simulink library "MathLib"  (R2016b)
settings: Solver=VariableStepAuto  StartTime=0.0  StopTime=10.0  RelTol=1e-3
settings Model: Creator=Administrator  LastModifiedBy=Administrator

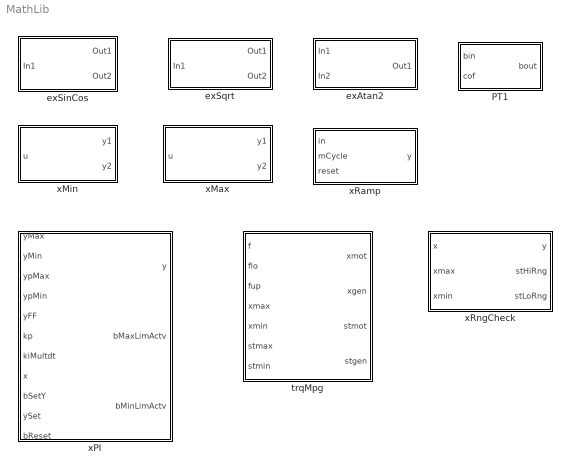
== system MathLib ==
  PT1 : Subsystem
      settings: RTWFcnNameOpts=Use subsystem name  RTWFileNameOpts=Use subsystem name
  exAtan2 : Subsystem
      mask help:
      | tan(theta) = yAxis/xAxis
      | theta: [0 65536) --> [0 360)
      mask Display:
      | disp('atan2 in C');
      | port_label('input',1,'yAxis');
      | port_label('input',2,'xAxis');
      | port_label('output',1,'theta');
  exSinCos : Subsystem
      mask help:
      | x: [0 65536) -->[0 360)
      | sin: [-32767 32767] -->[-1 1]
      | cos: [-32767 32767] -->[-1 1]
      mask Display:
      | disp('sincos in C');
      | port_label('input',1,'x');
      | port_label('output',1,'sinx');
      | port_label('output',2,'cosx');
  exSqrt : Subsystem
      mask help: x=0 when x<0
      mask Display:
      | disp('sqrt in C');
      | port_label('input',1,'x');
      | port_label('output',1,'sqrtx');
      | port_label('output',2,'1/sqrtx');
  trqMpg : MATLAB Function  TreatAsAtomicUnit=on
  xMax : MATLAB Function  TreatAsAtomicUnit=on
  xMin : MATLAB Function  TreatAsAtomicUnit=on
  xPI : MATLAB Function  TreatAsAtomicUnit=on
  xRamp : MATLAB Function  TreatAsAtomicUnit=on
  xRngCheck : MATLAB Function  TreatAsAtomicUnit=on

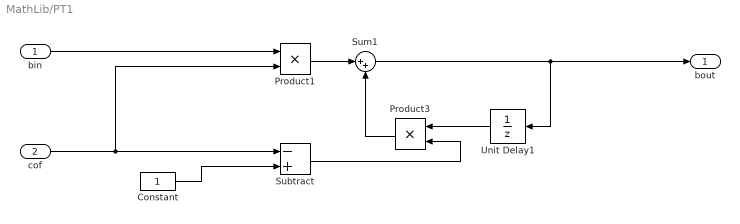
== system MathLib/PT1 ==
  bin : Inport
  cof : Inport  Port=2
  Constant : Constant  OutDataTypeStr=single
  Product1 : Product  RndMeth=Zero  OutDataTypeStr=Inherit: Same as first input
  Product3 : Product  RndMeth=Zero  OutDataTypeStr=Inherit: Same as first input
  Subtract : Sum  Inputs=-+  OutDataTypeStr=Inherit: Same as first input
  Sum1 : Sum  Inputs=|++  OutDataTypeStr=Inherit: Same as first input
  Unit Delay1 : UnitDelay  SampleTime=-1
  bout : Outport
  wires:
  Subtract/1 -> Product3/2
  Sum1/1 -> Unit Delay1/1, bout/1
  cof/1 -> Product1/2, Subtract/1
  Constant/1 -> Subtract/2
  bin/1 -> Product1/1
  Product1/1 -> Sum1/1
  Unit Delay1/1 -> Product3/1
  Product3/1 -> Sum1/2

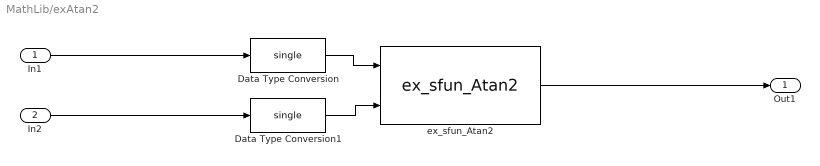
== system MathLib/exAtan2 ==
  In1 : Inport
  In2 : Inport  Port=2
  Data Type Conversion : DataTypeConversion  OutDataTypeStr=single
  Data Type Conversion1 : DataTypeConversion  OutDataTypeStr=single
  ex_sfun_Atan2 : S-Function  FunctionName=ex_sfun_Atan2  SFunctionDeploymentMode=off  EnableBusSupport=off  mask(Legacy Function){SFunctionSpec=void Atan2Shell(single u1,single u2,uint16 y1[1]), ShowSpec=on}
      mask prompts: ShowSpec "Display function specification"
      mask help:
      | This block allows you to call the legacy functions specified by the following Legacy Code Tool definition:
      | def.SFunctionName = 'ex_sfun_Atan2';
      | def.OutputFcnSpec = 'void Atan2Shell(single u1,single u2,uint16 y1[1])';
      | def.HeaderFiles = {'C2SfunShell.h', 'typedefs.h', 'LIB_Atan2.h', 'LIB_SinCosCalc.h', 'LIB_SqrtCalc.h'};
      | def.SourceFiles = {'C2SfunShell.c', 'LIB_Atan2.c', 'LIB_SinCosCalc.c', 'LIB_SqrtCalc.c'};
      mask Help: <p>This block was generated automatically by the Legacy Code Tool. For detailed help on this tool, call<a href="matlab:legacy_code('help')"> legacy_code('help')</a>.</p>
      mask Callback ShowSpec:
      | if strcmp(get_param(gcbh, 'ShowSpec'), 'on')
      |   set_param(gcbh, 'MaskDisplay', sprintf('fprintf(''%s'');', get_param(gcbh, 'SFunctionSpec')));
      | else
      |   set_param(gcbh, 'MaskDisplay', sprintf('fprintf(''%s'');', get_param(gcbh, 'FunctionName')));
      | end
      mask Display: fprintf('void Atan2Shell(single u1,single u2,uint16 y1[1])');
  Out1 : Outport
  wires:
  Data Type Conversion1/1 -> ex_sfun_Atan2/2
  Data Type Conversion/1 -> ex_sfun_Atan2/1
  In1/1 -> Data Type Conversion/1
  ex_sfun_Atan2/1 -> Out1/1
  In2/1 -> Data Type Conversion1/1

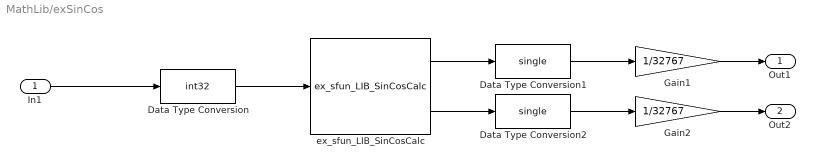
== system MathLib/exSinCos ==
  In1 : Inport
  Data Type Conversion : DataTypeConversion  OutDataTypeStr=int32
  Data Type Conversion1 : DataTypeConversion  OutDataTypeStr=single
  Data Type Conversion2 : DataTypeConversion  OutDataTypeStr=single
  Gain1 : Gain  Gain=1/32767
  Gain2 : Gain  Gain=1/32767
  ex_sfun_LIB_SinCosCalc : S-Function  FunctionName=ex_sfun_LIB_SinCosCalc  SFunctionDeploymentMode=off  EnableBusSupport=off  mask(Legacy Function){SFunctionSpec=void SinCosShell(int32 u1,int16 y1[1],int16 y2[1]), ShowSpec=on}
      mask prompts: ShowSpec "Display function specification"
      mask help:
      | This block allows you to call the legacy functions specified by the following Legacy Code Tool definition:
      | def.SFunctionName = 'ex_sfun_LIB_SinCosCalc';
      | def.OutputFcnSpec = 'void SinCosShell(int32 u1,int16 y1[1],int16 y2[1])';
      | def.HeaderFiles = {'C2SfunShell.h', 'typedefs.h', 'LIB_Atan2.h', 'LIB_SinCosCalc.h', 'LIB_SqrtCalc.h'};
      | def.SourceFiles = {'C2SfunShell.c', 'LIB_Atan2.c', 'LIB_SinCosCalc.c', 'LIB_SqrtCalc.c'};
      mask Help: <p>This block was generated automatically by the Legacy Code Tool. For detailed help on this tool, call<a href="matlab:legacy_code('help')"> legacy_code('help')</a>.</p>
      mask Callback ShowSpec:
      | if strcmp(get_param(gcbh, 'ShowSpec'), 'on')
      |   set_param(gcbh, 'MaskDisplay', sprintf('fprintf(''%s'');', get_param(gcbh, 'SFunctionSpec')));
      | else
      |   set_param(gcbh, 'MaskDisplay', sprintf('fprintf(''%s'');', get_param(gcbh, 'FunctionName')));
      | end
      mask Display: fprintf('void SinCosShell(int32 u1,int16 y1[1],int16 y2[1])');
  Out1 : Outport
  Out2 : Outport  Port=2
  wires:
  Gain1/1 -> Out1/1
  ex_sfun_LIB_SinCosCalc/1 -> Data Type Conversion1/1
  Data Type Conversion1/1 -> Gain1/1
  Data Type Conversion/1 -> ex_sfun_LIB_SinCosCalc/1
  In1/1 -> Data Type Conversion/1
  Data Type Conversion2/1 -> Gain2/1
  Gain2/1 -> Out2/1
  ex_sfun_LIB_SinCosCalc/2 -> Data Type Conversion2/1

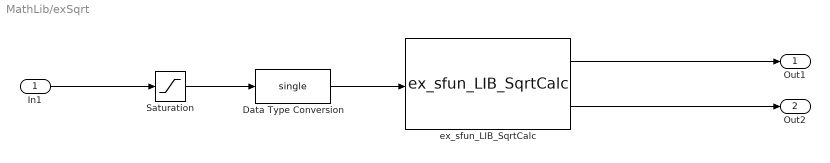
== system MathLib/exSqrt ==
  In1 : Inport
  Data Type Conversion : DataTypeConversion  OutDataTypeStr=single
  Saturation : Saturate  UpperLimit=inf  LowerLimit=0
  ex_sfun_LIB_SqrtCalc : S-Function  FunctionName=ex_sfun_LIB_SqrtCalc  SFunctionDeploymentMode=off  EnableBusSupport=off  mask(Legacy Function){SFunctionSpec=void SqrtShell(single u1,single y1[1],single y2[1]), ShowSpec=on}
      mask prompts: ShowSpec "Display function specification"
      mask help:
      | This block allows you to call the legacy functions specified by the following Legacy Code Tool definition:
      | def.SFunctionName = 'ex_sfun_LIB_SqrtCalc';
      | def.OutputFcnSpec = 'void SqrtShell(single u1,single y1[1],single y2[1])';
      | def.HeaderFiles = {'C2SfunShell.h', 'typedefs.h', 'LIB_Atan2.h', 'LIB_SinCosCalc.h', 'LIB_SqrtCalc.h'};
      | def.SourceFiles = {'C2SfunShell.c', 'LIB_Atan2.c', 'LIB_SinCosCalc.c', 'LIB_SqrtCalc.c'};
      mask Help: <p>This block was generated automatically by the Legacy Code Tool. For detailed help on this tool, call<a href="matlab:legacy_code('help')"> legacy_code('help')</a>.</p>
      mask Callback ShowSpec:
      | if strcmp(get_param(gcbh, 'ShowSpec'), 'on')
      |   set_param(gcbh, 'MaskDisplay', sprintf('fprintf(''%s'');', get_param(gcbh, 'SFunctionSpec')));
      | else
      |   set_param(gcbh, 'MaskDisplay', sprintf('fprintf(''%s'');', get_param(gcbh, 'FunctionName')));
      | end
      mask Display: fprintf('void SqrtShell(single u1,single y1[1],single y2[1])');
  Out1 : Outport
  Out2 : Outport  Port=2
  wires:
  ex_sfun_LIB_SqrtCalc/2 -> Out2/1
  In1/1 -> Saturation/1
  ex_sfun_LIB_SqrtCalc/1 -> Out1/1
  Data Type Conversion/1 -> ex_sfun_LIB_SqrtCalc/1
  Saturation/1 -> Data Type Conversion/1

== matlab function MathLib/xMax ==
  data: u input; y1 output; y2 output
function [y1,y2] = xMax(u)

[y1,y2] = max(u);

end

== matlab function MathLib/xMin ==
  data: u input; y1 output; y2 output
function [y1,y2] = xMin(u)

[y1,y2] = min(u);

end

== matlab function MathLib/trqMpg ==
  data: f input; flo input; fup input; xmot output; xmax input; xmin input; stmax input; stmin input; xgen output; stmot output; stgen output
function [xmot,xgen,stmot,stgen] = trqMappping(f,flo,fup,xmax, xmin, stmax,stmin)

% change from xmax(-flo) to -xmin(-fup)
if f>=(-flo)
    xmot = xmax;
    stmot = stmax;
else if f<=(-fup)
        xmot = -xmin;
        stmot = stmin;
    else
        xmot = (f-(-flo))/((-fup)-(-flo))*((-xmin)-xmax)+xmax;
        stmot = stmax;
    end
end
% change from xmin(fup) to -xmax(flo)
if f>= fup
    xgen = xmin;
    stgen = stmin;
else if f<=flo
        xgen = -xmax;
        stgen = stmax;
    else
        xgen = (f-fup)/(flo-fup)*((-xmax)-xmin)+xmin;
        stgen = stmin;
    end
end
end

== matlab function MathLib/xPI ==
  data: yMax input; yMin input; ypMax input; y output; ypMin input; yFF input; kp input; kiMultdt input; x input; bSetY input; ySet input; bReset input; bMaxLimActv output; bMinLimActv output
function [y,bMaxLimActv,bMinLimActv] = xPI(yMax,yMin,ypMax,ypMin,yFF,kp,kiMultdt,x,bSetY,ySet,bReset)
persistent yi;
if isempty(yi)
    yi = single(0);
end

if bReset
    bMaxLimActv = false;
    bMinLimActv = false;
    yi = single(0);
    y = single(0);
else
     yiAdd = kiMultdt*x;
     yp = max(min(kp*x, ypMax),ypMin);	
     ypSumyFF = yp + yFF;
     if bSetY					% set output: y = ySet	
     	yi = ySet - ypSumyFF - yiAdd;
     end
     
      yiNew = yiAdd + yi;
      yUnlim = yiNew + ypSumyFF;
 
     if (yUnlim >= yMax) 		% controller limited by yMax
     	bMaxLimActv = true;
        bMinLimActv = false;
     	y = yMax;
     	yi = max((yMax - ypSumyFF), 0);
    else if(yUnlim <= yMin)     % controller limited by yMin
            bMaxLimActv = false;
            bMinLimActv = true;
        	y = yMin;
        	yi = min((yMin - ypSumyFF), 0);
           else                       % controller not limited
         	bMaxLimActv = false;
        	bMinLimActv = false;
        	y = (yUnlim);
        	yi = (yiNew);
           end
     end
end

end

== matlab function MathLib/xRamp ==
  data: in input; y output; mCycle input; reset input
function y = xRamp(in,mCycle,reset)
persistent out;
if isempty(out)
    out = single(0);
end

if (reset) 
	out = in;
else                        % Reset condition ramp off
	dy = in - out;			% determine the maximum possible jump
	mCycleTmp = mCycle;		% only one push operator is required
	dy = min(mCycleTmp, dy);	% Limit the jump by increasing the slope
	dy = max(-mCycleTmp,dy);    % Limit the jump by downward slope
	out = (out + dy);           %  Jump to output.
end

y=out;
end

== matlab function MathLib/xRngCheck ==
  data: x input; xmax input; y output; xmin input; stHiRng output; stLoRng output
function [y, stHiRng, stLoRng] = xRngCheck(x, xmax,xmin)

persistent out;
if isempty(out)
    out = single(0);
end

if x>xmax
    stHiRng = true;
    stLoRng = false;
    out = xmax;
elseif x< xmin
    stLoRng = true;
    stHiRng = false;
    out = xmin;
else
    out = x;
    stLoRng = false;
    stHiRng = false;
end

y = out;
